simulink library "inp"  (R2021b)
settings: Solver=VariableStepAuto  StartTime=0.0  StopTime=10.0  RelTol=1e-3
undefined symbols (not defined in the file): C_TASK_5MS_S, FALSE, KINP_AcoreReadyToSlp_flg_ovrdflg, KINP_AcoreReadyToSlp_flg_ovrdval, KINP_AllowMovThd_OTA_enum_ovrdflg, KINP_AllowMovThd_OTA_enum_ovrdval, KINP_APSAngleTarget_Deg_ovrdflg, KINP_APSAngleTarget_Deg_ovrdval, KINP_APSDecReq_mps2_ovrdflg, KINP_APSDecReq_mps2_ovrdval, KINP_APSDecReqA_flg_ovrdflg, KINP_APSDecReqA_flg_ovrdval, KINP_APSDFLL_cm_ovrdflg, KINP_APSDFLL_cm_ovrdval, KINP_APSDFLR_cm_ovrdflg, KINP_APSDFLR_cm_ovrdval, KINP_APSDRLL_cm_ovrdflg, KINP_APSDRLL_cm_ovrdval, KINP_APSDRLR_cm_ovrdflg, KINP_APSDRLR_cm_ovrdval, KINP_APSExitCondition_enum_ovrdflg, KINP_APSExitCondition_enum_ovrdval, KINP_APSHWVer_enum_ovrdflg, KINP_APSHWVer_enum_ovrdval, KINP_APSProgressPCT_pct_ovrdflg, KINP_APSProgressPCT_pct_ovrdval, KINP_APSPwrReq_enum_ovrdflg, KINP_APSPwrReq_enum_ovrdval, KINP_APSReq_enum_ovrdflg, KINP_APSReq_enum_ovrdval, KINP_APSRQDisplay_enum_ovrdflg, KINP_APSRQDisplay_enum_ovrdval, KINP_APSRqEPASCtrl_flg_ovrdflg, KINP_APSRqEPASCtrl_flg_ovrdval, KINP_APSShiftPosnReq_enum_ovrdval, KINP_APSShiftPosnReq_enum_ovrflg, KINP_APSSpeedCMD_kph_ovrdval, KINP_APSSpeedCMD_kph_ovrflg, KINP_APSStaSystem_enum_ovrdflg, KINP_APSStaSystem_enum_ovrdval, KINP_APSSWVer_enum_ovrdflg, KINP_APSSWVer_enum_ovrdval, KINP_APSVMCReqA_flg_ovrdval, KINP_APSVMCReqA_flg_ovrflg, KINP_APSVRqEPASCtrl_flg_ovrdflg, KINP_APSVRqEPASCtrl_flg_ovrdval, KINP_AuxBattVolmV_mV_ovrdflg, KINP_AuxBattVolmV_mV_ovrdval, KINP_CAASSta_enum_ovrdflg, KINP_CAASSta_enum_ovrdval, KINP_CAASVMCReqA_flg_ovrdval, KINP_CAASVMCReqA_flg_ovrflg, KINP_CAN1BusOff_flg_ovrdflg, KINP_CAN1BusOff_flg_ovrdval, KINP_CAN2BusOff_flg_ovrdflg, KINP_CAN2BusOff_flg_ovrdval, KINP_CAN3BusOff_flg_ovrdflg, KINP_CAN3BusOff_flg_ovrdval, KINP_CAN4BusOff_flg_ovrdflg, KINP_CAN4BusOff_flg_ovrdval ... (+152)
libraries: FVT_lib x1037, hcu_lib x1
(part 7 of 34)

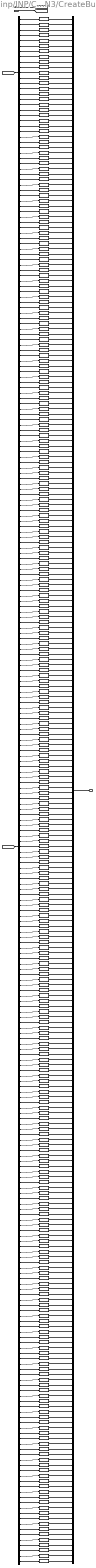
== system inp/INP/CAN3/CreateBus ==
  inp_CanValid_bus : Inport
  inp_Hal_bus : Inport  Port=2
  UnitConverter_{1..23,35,44,63..64,67..75,81..83,87,91..92,102,104..105,107,109,113,115..116,123..125,132..133,135..137,162..164,171..172,174..176,197..201,210..211,213..215,237..238,240..242,251..252,254..256,277..278,283..285,288} (92 alike) : DataTypeConversion  OutDataTypeStr=boolean
  UnitConverter_{26..34,36..43,45..53,58..62,94..97,99..100,110..112,117,126,128..131,139..145,147..148,153..154,161,165,167..170,178..184,186,191..192,202,204,207..209,217..223,225..226,231..232,243,245,248..250,258..266,271..272} (105 alike) : DataTypeConversion  OutDataTypeStr=single
  UnitConverter_{24..25,54..57,65..66,76..80,84..86,88..90,93,98,101,103,106,108,114,118..122,127,134,138,146,149..152,155,158..160,166,173,177,185,187..190,195..196,203,205..206,212,216,224,227..230,233..234,239,244,246..247,253,257,267..270,273..274,279..282,286..287,289..290} (85 alike) : DataTypeConversion  OutDataTypeStr=uint8
  UnitConverter_{156..157,193..194,235..236,275..276} (8 alike) : DataTypeConversion  OutDataTypeStr=uint16
  bus_creator : BusCreator  Inputs=290
  bus_selector : BusSelector  OutputSignals=VINP_CANMsgValidBMS1_flg,VINP_CANMsgValidBMS3_flg,VINP_CANMsgValidBMS4_flg,VINP_CANMsgValidBMS5_flg,VINP_CANMsgValidBMS6_flg,VINP_CANMsgValidBMS8_flg,VINP_CANMsgValidCCU1_flg,VINP_CANMsgValidCCU2_flg,VINP_CANMsgValidEBM1_flg,VINP_CANMsgValidMCUBF1_flg,VINP_CANMsgValidMCUBF2_flg,VINP_CANMsgValidMCUBR1_flg,VINP_CANMsgValidMCUBR2_flg,VINP_CANMsgValidMCUNF1_flg,VINP_CANMsgValidMCUNF2_flg,VINP_CANMsgValidMCUNF3_flg,VINP_CANMsgValidMCUNR1_flg,VINP_CANMsgValidMCUNR2_flg,VINP_CANMsgValidMCUNR3_flg,VINP_CANMsgValidShifter1_flg,VINP_CANMsgValidShifter2_flg
  bus_selector_1 : BusSelector  OutputSignals=VINP_BMS1CSErr_flg,VINP_BMS1RCErr_flg,VINP_BMSChckSum1_enum,VINP_BMSRolCnct1_enum,VINP_HVBPwrAvailChrg_kW,VINP_HVBPwrAvailChrg30_kW,VINP_HVBPwrAvailChrg60_kW,VINP_HVBPwrAvailDchrg_kW,VINP_HVBPwrAvailDchrg30_kW,VINP_HVBPwrAvailDchrg60_kW,VINP_HVBattCurr_A,VINP_HVBattVolt_V,VINP_ACChrgCurrDis_A,VINP_FireDetErr_flg,VINP_HVBChrgPwr_kWh,VINP_HVBChrgPwrTotal_kWh,VINP_HVBDrvPwr_kWh,VINP_HVBDrvPwrTotal_kWh,VINP_HVBFullChrgPwr_kWh,VINP_HVBIsoImpedenceN_Megaohm,VINP_HVBIsoImpedenceP_Megaohm,VINP_HVBSOH_pct,VINP_HVBattErr_flg,VINP_HVBattPackVolt_V,VINP_HVBattSOC_pct,VINP_HVBattSOCDis_pct,VINP_RemainChrgTime_min,VINP_CellTempAvg_C,VINP_HVBCellVoltMax_mV,VINP_HVBCellVoltMin_mV,VINP_HVBMTempMax_C,VINP_HVBMTempMin_C,VINP_MaxCellTempNum_enum,VINP_MaxCellVoltNum_enum,VINP_MinCellTempNum_enum,VINP_MinCellVoltNum_enum,VINP_HVInVolt_V,VINP_LVBattDet12V_V,VINP_OBCACCSLimit_A,VINP_OBCDCCurLm_A,VINP_OBCDCVoltLm_V,VINP_BMS6CSErr_flg,VINP_BMS6RCErr_flg,VINP_BMSChckSum_enum,VINP_BMSRolCnct_enum,VINP_BMSREADY_flg,VINP_BMSWarn1_flg,VINP_BMSWarn2_flg,VINP_BMSWarn3_flg,VINP_BMSWarn4_flg,VINP_BMSWarn5_flg,VINP_BMSWarn6_flg,VINP_BMSWarn7_flg,VINP_BMSWarn8_flg,VINP_ChrgInLockReq_enum,VINP_ChrgPlugSta_enum,VINP_DisChrgPlugErr_enum,VINP_ExtChrgSta_enum,VINP_HVBChrgErr_enum,VINP_HVBContactorSta_flg,VINP_HVBHVILErr_flg,VINP_HVBOvrTempErr_flg,VINP_HVBOvrTempWarn_enum,VINP_HVBPreheatPrecoolSta_enum,VINP_HVBattReady4Pre_enum,VINP_HVILSta_flg,VINP_V2LSta_enum,VINP_MainRlyNegSta_enum,VINP_MainRlyPosSta_enum,VINP_CCU1CSErr_flg,VINP_CCU1RCErr_flg,VINP_CSCCU1_enum,VINP_DCDCAuxCur_A,VINP_DCDCAuxVolt_V,VINP_DCDCHVCur_A,VINP_DCDCInVoltInf_V,VINP_DCDCPreCompleted_enum,VINP_OBCDCCurrInf_A,VINP_OBCDCVoltInf_V,VINP_OBCPreCompleted_enum,VINP_OBCWakeup4Plugin_flg,VINP_RCCCU1_enum,VINP_CCU2CSErr_flg,VINP_CCU2RCErr_flg,VINP_CSCCU2_enum,VINP_DCDCEnaSta_flg,VINP_DCDCFaultSta_enum,VINP_DCDCReady4Pre_flg,VINP_DCDCTemp_C,VINP_OBCACCurrInf_A,VINP_OBCACVoltInf_V,VINP_OBCEnaSta_flg,VINP_OBCFaultSta_enum,VINP_OBCPluginSta_flg,VINP_OBCReady4Pre_flg,VINP_OBCTemp_C,VINP_OBCV2LSta_enum,VINP_OBCACCurLim_enum,VINP_RCCCU2_enum,VINP_EBMErrSta_enum,VINP_EBMRLampSta_enum,VINP_FrActvDmpDisabSta_flg,VINP_FrEDUDrtSta_flg,VINP_FrEDUOpratingSta_flg,VINP_FrEDURealTMTq_Nm,VINP_FrEDURotateDirction_enum,VINP_FrEDUTqReqFbk_Nm,VINP_FrMCUBAT_V,VINP_FrMCUDCBusCurr_A,VINP_FrMCUDCBusVolt_V,VINP_FrMCUDischrgSta_flg,VINP_FrMCUEnaSta_flg,VINP_FrMCUErr_enum,VINP_FrMCUIGNsta_flg,VINP_FrMCUReady_flg,VINP_FrMCUReady4Pre_flg,VINP_FrMCUSysSta_enum,VINP_FrMCUTemp_C,VINP_FrMotorAvailTq_Nm,VINP_FrRegenAvailTq_Nm,VINP_FrTMSpd_rpm,VINP_FrTMTemp_C,VINP_FrTMid_A,VINP_FrTMiq_A,VINP_MCUWarnF_enum,VINP_MCUBFRealPwrKwSta_kW,VINP_FrCoolanttempReq_C,VINP_FrFailcode1_enum,VINP_FrFailcode2_enum,VINP_FrFailcodehistory1_enum,VINP_FrFailcodehistory2_enum,VINP_FrLLCTemp_C,VINP_FrLLCflowReq_Lpmin,VINP_FrMCUTempWarn_enum,VINP_FrMCUHWVer_enum,VINP_FrMCUSWVer_enum,VINP_FrTMTempWarn_enum,VINP_MCUBFLLCTempWarnSta_enum,VINP_MCUWarnR_enum,VINP_MCUBRRealPwrKwSta_kW,VINP_RrActvDmpDisabSta_flg,VINP_RrEDUDrtSta_flg,VINP_RrEDUOpratingSta_flg,VINP_RrEDURealTMTq_Nm,VINP_RrEDURotateDirction_enum,VINP_RrEDUTqReqFbk_Nm,VINP_RrMCUBAT_V,VINP_RrMCUDCBusCurr_A,VINP_RrMCUDCBusVolt_V,VINP_RrMCUDischrgSta_flg,VINP_RrMCUEnaSta_flg,VINP_RrMCUErr_enum,VINP_RrMCUIGNsta_flg,VINP_RrMCUReady_flg,VINP_RrMCUReady4Pre_flg,VINP_RrMCUSysSta_enum,VINP_RrMCUTemp_C,VINP_RrMotorAvailTq_Nm,VINP_RrRegenAvailTq_Nm,VINP_RrTMSpd_rpm,VINP_RrTMTemp_C,VINP_RrTMid_A,VINP_RrTMiq_A,VINP_MCUBRLLCTempWarnSta_enum,VINP_RrCoolanttempReq_cnt,VINP_RrFailcode1_enum,VINP_RrFailcode2_enum,VINP_RrFailcodehistory1_enum,VINP_RrFailcodehistory2_enum,VINP_RrLLCTemp_C,VINP_RrLLCflowReq_Lpmin,VINP_RrMCU3HWVer_enum,VINP_RrMCU3SWVer_enum,VINP_RrMCUTempWarn_enum,VINP_RrTMTempWarn_enum,VINP_MCUNF1CSErr_flg,VINP_MCUNF1RCErr_flg,VINP_FrActvDmpDisabStaNidec_flg,VINP_FrEDUDrtStaNidec_flg,VINP_FrEDUOpratingStaNidec_flg,VINP_FrEDURealTMTqNidec_Nm,VINP_FrEDURotateDirctionNidec_enum,VINP_FrEDUTqReqFbkNidec_Nm,VINP_FrMCU1ChksumNidec_enum,VINP_FrMCU1RolCntNidec_enum,VINP_FrMCUBATNidec_V,VINP_FrMCUDCBusCurrNidec_A,VINP_FrMCUDCBusVoltNidec_V,VINP_FrMCUDischrgStaNidec_flg,VINP_FrMCUEnaStaNidec_flg,VINP_FrMCUErrNidec_enum,VINP_FrMCUIGNstaNidec_flg,VINP_FrMCUReady4PreNidec_flg,VINP_FrMCUReadyNidec_flg,VINP_FrMCUSysStaNidec_enum,VINP_FrMCUTempNidec_C,VINP_FrMotorAvailTqNidec_Nm,VINP_FrRegenAvailTqNidec_Nm,VINP_FrTMSpdNidec_rpm,VINP_FrTMTempNidec_C,VINP_FrTMidNidec_A,VINP_FrTMiqNidec_A,VINP_MCUWarnFNidec_enum,VINP_FrCoolanttempReqNidec_C,VINP_FrEOPSpdSetNidec_rpm,VINP_FrFailcode1Nidec_enum,VINP_FrFailcode2Nidec_enum,VINP_FrFailcodehistory1Nidec_enum,VINP_FrFailcodehistory2Nidec_enum,VINP_FrLLCTempNidec_C,VINP_FrLLCflowReqNidec_Lpmin,VINP_FrMCUTempWarnNidec_enum,VINP_FrTMTempWarnNidec_enum,VINP_FrMCUHWVerNidec_enum,VINP_FrMCUSWVerNidec_enum,VINP_MCUNR1CSErr_flg,VINP_MCUNR1RCErr_flg,VINP_MCUWarnRNidec_enum,VINP_RrActvDmpDisabStaNidec_flg,VINP_RrEDUDrtStaNidec_flg,VINP_RrEDUOpratingStaNidec_flg,VINP_RrEDURealTMTqNidec_Nm,VINP_RrEDURotateDirctionNidec_enum,VINP_RrEDUTqReqFbkNidec_Nm,VINP_RrMCU1ChksumNidec_enum,VINP_RrMCU1RolCntNidec_enum,VINP_RrMCUBATNidec_V,VINP_RrMCUDCBusCurrNidec_A,VINP_RrMCUDCBusVoltNidec_V,VINP_RrMCUDischrgStaNidec_flg,VINP_RrMCUEnaStaNidec_flg,VINP_RrMCUErrNidec_enum,VINP_RrMCUIGNstaNidec_flg,VINP_RrMCUReady4PreNidec_flg,VINP_RrMCUReadyNidec_flg,VINP_RrMCUSysStaNidec_enum,VINP_RrMCUTempNidec_C,VINP_RrMotorAvailTqNidec_Nm,VINP_RrRegenAvailTqNidec_Nm,VINP_RrTMSpdNidec_rpm,VINP_RrTMTempNidec_C,VINP_RrTMidNidec_A,VINP_RrTMiqNidec_A,VINP_RrCoolanttempReqNidec_cnt,VINP_RrEOPSpdSetNidec_rpm,VINP_RrFailcode1Nidec_enum,VINP_RrFailcode2Nidec_enum,VINP_RrFailcodehistory1Nidec_enum,VINP_RrFailcodehistory2Nidec_enum,VINP_RrLLCTempNidec_C,VINP_RrLLCflowReqNidec_Lpmin,VINP_RrMCUTempWarnNidec_enum,VINP_RrTMTempWarnNidec_enum,VINP_RrMCU3HWVerNidec_enum,VINP_RrMCU3SWVerNidec_enum,VINP_Shifter1CSErr_flg,VINP_Shifter1RCErr_flg,VINP_ShifterCRC8_enum,VINP_ShifterFailsta_enum,VINP_ShifterHandleCmd_enum,VINP_ShifterRC_enum,VINP_Shifter2CSErr_flg,VINP_Shifter2RCErr_flg,VINP_CSW2DimSwSta_flg,VINP_CSW2FWasSwSta_enum,VINP_CSW2FWipSwSta_enum,VINP_CSW2PassSWSta_flg,VINP_CSW2RWipWasSwSta_enum,VINP_CSW2TurnSwSta_enum
  BINP_outputs : Outport
  wires:
  inp_CanValid_bus/1 -> [inp_CanValid_bus]
  inp_Hal_bus/1 -> [inp_Hal_bus]
  bus_selector/1 -> UnitConverter_1/1  "<VINP_CANMsgValidBMS1_flg>"
  UnitConverter_1/1 -> bus_creator/1  "VINP_CANMsgValidBMS1_flg"
  bus_selector/2 -> UnitConverter_2/1  "<VINP_CANMsgValidBMS3_flg>"
  UnitConverter_2/1 -> bus_creator/2  "VINP_CANMsgValidBMS3_flg"
  bus_selector/3 -> UnitConverter_3/1  "<VINP_CANMsgValidBMS4_flg>"
  UnitConverter_3/1 -> bus_creator/3  "VINP_CANMsgValidBMS4_flg"
  bus_selector/4 -> UnitConverter_4/1  "<VINP_CANMsgValidBMS5_flg>"
  UnitConverter_4/1 -> bus_creator/4  "VINP_CANMsgValidBMS5_flg"
  bus_selector/5 -> UnitConverter_5/1  "<VINP_CANMsgValidBMS6_flg>"
  UnitConverter_5/1 -> bus_creator/5  "VINP_CANMsgValidBMS6_flg"
  bus_selector/6 -> UnitConverter_6/1  "<VINP_CANMsgValidBMS8_flg>"
  UnitConverter_6/1 -> bus_creator/6  "VINP_CANMsgValidBMS8_flg"
  bus_selector/7 -> UnitConverter_7/1  "<VINP_CANMsgValidCCU1_flg>"
  UnitConverter_7/1 -> bus_creator/7  "VINP_CANMsgValidCCU1_flg"
  bus_selector/8 -> UnitConverter_8/1  "<VINP_CANMsgValidCCU2_flg>"
  UnitConverter_8/1 -> bus_creator/8  "VINP_CANMsgValidCCU2_flg"
  bus_selector/9 -> UnitConverter_9/1  "<VINP_CANMsgValidEBM1_flg>"
  UnitConverter_9/1 -> bus_creator/9  "VINP_CANMsgValidEBM1_flg"
  bus_selector/10 -> UnitConverter_10/1  "<VINP_CANMsgValidMCUBF1_flg>"
  UnitConverter_10/1 -> bus_creator/10  "VINP_CANMsgValidMCUBF1_flg"
  bus_selector/11 -> UnitConverter_11/1  "<VINP_CANMsgValidMCUBF2_flg>"
  UnitConverter_11/1 -> bus_creator/11  "VINP_CANMsgValidMCUBF2_flg"
  bus_selector/12 -> UnitConverter_12/1  "<VINP_CANMsgValidMCUBR1_flg>"
  UnitConverter_12/1 -> bus_creator/12  "VINP_CANMsgValidMCUBR1_flg"
  bus_selector/13 -> UnitConverter_13/1  "<VINP_CANMsgValidMCUBR2_flg>"
  UnitConverter_13/1 -> bus_creator/13  "VINP_CANMsgValidMCUBR2_flg"
  bus_selector/14 -> UnitConverter_14/1  "<VINP_CANMsgValidMCUNF1_flg>"
  UnitConverter_14/1 -> bus_creator/14  "VINP_CANMsgValidMCUNF1_flg"
  bus_selector/15 -> UnitConverter_15/1  "<VINP_CANMsgValidMCUNF2_flg>"
  UnitConverter_15/1 -> bus_creator/15  "VINP_CANMsgValidMCUNF2_flg"
  bus_selector/16 -> UnitConverter_16/1  "<VINP_CANMsgValidMCUNF3_flg>"
  UnitConverter_16/1 -> bus_creator/16  "VINP_CANMsgValidMCUNF3_flg"
  bus_selector/17 -> UnitConverter_17/1  "<VINP_CANMsgValidMCUNR1_flg>"
  UnitConverter_17/1 -> bus_creator/17  "VINP_CANMsgValidMCUNR1_flg"
  bus_selector/18 -> UnitConverter_18/1  "<VINP_CANMsgValidMCUNR2_flg>"
  UnitConverter_18/1 -> bus_creator/18  "VINP_CANMsgValidMCUNR2_flg"
  bus_selector/19 -> UnitConverter_19/1  "<VINP_CANMsgValidMCUNR3_flg>"
  UnitConverter_19/1 -> bus_creator/19  "VINP_CANMsgValidMCUNR3_flg"
  bus_selector/20 -> UnitConverter_20/1  "<VINP_CANMsgValidShifter1_flg>"
  UnitConverter_20/1 -> bus_creator/20  "VINP_CANMsgValidShifter1_flg"
  bus_selector/21 -> UnitConverter_21/1  "<VINP_CANMsgValidShifter2_flg>"
  UnitConverter_21/1 -> bus_creator/21  "VINP_CANMsgValidShifter2_flg"
  bus_selector_1/1 -> UnitConverter_22/1  "<VINP_BMS1CSErr_flg>"
  UnitConverter_22/1 -> bus_creator/22  "VINP_BMS1CSErr_flg"
  bus_selector_1/2 -> UnitConverter_23/1  "<VINP_BMS1RCErr_flg>"
  UnitConverter_23/1 -> bus_creator/23  "VINP_BMS1RCErr_flg"
  bus_selector_1/3 -> UnitConverter_24/1  "<VINP_BMSChckSum1_enum>"
  UnitConverter_24/1 -> bus_creator/24  "VINP_BMSChckSum1_enum"
  bus_selector_1/4 -> UnitConverter_25/1  "<VINP_BMSRolCnct1_enum>"
  UnitConverter_25/1 -> bus_creator/25  "VINP_BMSRolCnct1_enum"
  bus_selector_1/5 -> UnitConverter_26/1  "<VINP_HVBPwrAvailChrg_kW>"
  UnitConverter_26/1 -> bus_creator/26  "VINP_HVBPwrAvailChrg_kW"
  bus_selector_1/6 -> UnitConverter_27/1  "<VINP_HVBPwrAvailChrg30_kW>"
  UnitConverter_27/1 -> bus_creator/27  "VINP_HVBPwrAvailChrg30_kW"
  bus_selector_1/7 -> UnitConverter_28/1  "<VINP_HVBPwrAvailChrg60_kW>"
  UnitConverter_28/1 -> bus_creator/28  "VINP_HVBPwrAvailChrg60_kW"
  bus_selector_1/8 -> UnitConverter_29/1  "<VINP_HVBPwrAvailDchrg_kW>"
  UnitConverter_29/1 -> bus_creator/29  "VINP_HVBPwrAvailDchrg_kW"
  bus_selector_1/9 -> UnitConverter_30/1  "<VINP_HVBPwrAvailDchrg30_kW>"
  UnitConverter_30/1 -> bus_creator/30  "VINP_HVBPwrAvailDchrg30_kW"
  bus_selector_1/10 -> UnitConverter_31/1  "<VINP_HVBPwrAvailDchrg60_kW>"
  UnitConverter_31/1 -> bus_creator/31  "VINP_HVBPwrAvailDchrg60_kW"
  bus_selector_1/11 -> UnitConverter_32/1  "<VINP_HVBattCurr_A>"
  UnitConverter_32/1 -> bus_creator/32  "VINP_HVBattCurr_A"
  bus_selector_1/12 -> UnitConverter_33/1  "<VINP_HVBattVolt_V>"
  UnitConverter_33/1 -> bus_creator/33  "VINP_HVBattVolt_V"
  bus_selector_1/13 -> UnitConverter_34/1  "<VINP_ACChrgCurrDis_A>"
  UnitConverter_34/1 -> bus_creator/34  "VINP_ACChrgCurrDis_A"
  bus_selector_1/14 -> UnitConverter_35/1  "<VINP_FireDetErr_flg>"
  UnitConverter_35/1 -> bus_creator/35  "VINP_FireDetErr_flg"
  bus_selector_1/15 -> UnitConverter_36/1  "<VINP_HVBChrgPwr_kWh>"
  UnitConverter_36/1 -> bus_creator/36  "VINP_HVBChrgPwr_kWh"
  bus_selector_1/16 -> UnitConverter_37/1  "<VINP_HVBChrgPwrTotal_kWh>"
  UnitConverter_37/1 -> bus_creator/37  "VINP_HVBChrgPwrTotal_kWh"
  bus_selector_1/17 -> UnitConverter_38/1  "<VINP_HVBDrvPwr_kWh>"
  UnitConverter_38/1 -> bus_creator/38  "VINP_HVBDrvPwr_kWh"
  bus_selector_1/18 -> UnitConverter_39/1  "<VINP_HVBDrvPwrTotal_kWh>"
  UnitConverter_39/1 -> bus_creator/39  "VINP_HVBDrvPwrTotal_kWh"
  bus_selector_1/19 -> UnitConverter_40/1  "<VINP_HVBFullChrgPwr_kWh>"
  UnitConverter_40/1 -> bus_creator/40  "VINP_HVBFullChrgPwr_kWh"
  bus_selector_1/20 -> UnitConverter_41/1  "<VINP_HVBIsoImpedenceN_Megaohm>"
  UnitConverter_41/1 -> bus_creator/41  "VINP_HVBIsoImpedenceN_Megaohm"
  bus_selector_1/21 -> UnitConverter_42/1  "<VINP_HVBIsoImpedenceP_Megaohm>"
  UnitConverter_42/1 -> bus_creator/42  "VINP_HVBIsoImpedenceP_Megaohm"
  bus_selector_1/22 -> UnitConverter_43/1  "<VINP_HVBSOH_pct>"
  UnitConverter_43/1 -> bus_creator/43  "VINP_HVBSOH_pct"
  bus_selector_1/23 -> UnitConverter_44/1  "<VINP_HVBattErr_flg>"
  UnitConverter_44/1 -> bus_creator/44  "VINP_HVBattErr_flg"
  bus_selector_1/24 -> UnitConverter_45/1  "<VINP_HVBattPackVolt_V>"
  UnitConverter_45/1 -> bus_creator/45  "VINP_HVBattPackVolt_V"
  bus_selector_1/25 -> UnitConverter_46/1  "<VINP_HVBattSOC_pct>"
  UnitConverter_46/1 -> bus_creator/46  "VINP_HVBattSOC_pct"
  bus_selector_1/26 -> UnitConverter_47/1  "<VINP_HVBattSOCDis_pct>"
  UnitConverter_47/1 -> bus_creator/47  "VINP_HVBattSOCDis_pct"
  bus_selector_1/27 -> UnitConverter_48/1  "<VINP_RemainChrgTime_min>"
  UnitConverter_48/1 -> bus_creator/48  "VINP_RemainChrgTime_min"
  bus_selector_1/28 -> UnitConverter_49/1  "<VINP_CellTempAvg_C>"
  UnitConverter_49/1 -> bus_creator/49  "VINP_CellTempAvg_C"
  bus_selector_1/29 -> UnitConverter_50/1  "<VINP_HVBCellVoltMax_mV>"
  UnitConverter_50/1 -> bus_creator/50  "VINP_HVBCellVoltMax_mV"
  bus_selector_1/30 -> UnitConverter_51/1  "<VINP_HVBCellVoltMin_mV>"
  UnitConverter_51/1 -> bus_creator/51  "VINP_HVBCellVoltMin_mV"
  bus_selector_1/31 -> UnitConverter_52/1  "<VINP_HVBMTempMax_C>"
  UnitConverter_52/1 -> bus_creator/52  "VINP_HVBMTempMax_C"
  bus_selector_1/32 -> UnitConverter_53/1  "<VINP_HVBMTempMin_C>"
  UnitConverter_53/1 -> bus_creator/53  "VINP_HVBMTempMin_C"
  bus_selector_1/33 -> UnitConverter_54/1  "<VINP_MaxCellTempNum_enum>"
  UnitConverter_54/1 -> bus_creator/54  "VINP_MaxCellTempNum_enum"
  bus_selector_1/34 -> UnitConverter_55/1  "<VINP_MaxCellVoltNum_enum>"
  UnitConverter_55/1 -> bus_creator/55  "VINP_MaxCellVoltNum_enum"
  bus_selector_1/35 -> UnitConverter_56/1  "<VINP_MinCellTempNum_enum>"
  UnitConverter_56/1 -> bus_creator/56  "VINP_MinCellTempNum_enum"
  bus_selector_1/36 -> UnitConverter_57/1  "<VINP_MinCellVoltNum_enum>"
  UnitConverter_57/1 -> bus_creator/57  "VINP_MinCellVoltNum_enum"
  bus_selector_1/37 -> UnitConverter_58/1  "<VINP_HVInVolt_V>"
  UnitConverter_58/1 -> bus_creator/58  "VINP_HVInVolt_V"
  bus_selector_1/38 -> UnitConverter_59/1  "<VINP_LVBattDet12V_V>"
  UnitConverter_59/1 -> bus_creator/59  "VINP_LVBattDet12V_V"
  bus_selector_1/39 -> UnitConverter_60/1  "<VINP_OBCACCSLimit_A>"
  UnitConverter_60/1 -> bus_creator/60  "VINP_OBCACCSLimit_A"
  bus_selector_1/40 -> UnitConverter_61/1  "<VINP_OBCDCCurLm_A>"
  UnitConverter_61/1 -> bus_creator/61  "VINP_OBCDCCurLm_A"
  bus_selector_1/41 -> UnitConverter_62/1  "<VINP_OBCDCVoltLm_V>"
  UnitConverter_62/1 -> bus_creator/62  "VINP_OBCDCVoltLm_V"
  bus_selector_1/42 -> UnitConverter_63/1  "<VINP_BMS6CSErr_flg>"
  UnitConverter_63/1 -> bus_creator/63  "VINP_BMS6CSErr_flg"
  bus_selector_1/43 -> UnitConverter_64/1  "<VINP_BMS6RCErr_flg>"
  UnitConverter_64/1 -> bus_creator/64  "VINP_BMS6RCErr_flg"
  bus_selector_1/44 -> UnitConverter_65/1  "<VINP_BMSChckSum_enum>"
  UnitConverter_65/1 -> bus_creator/65  "VINP_BMSChckSum_enum"
  bus_selector_1/45 -> UnitConverter_66/1  "<VINP_BMSRolCnct_enum>"
  UnitConverter_66/1 -> bus_creator/66  "VINP_BMSRolCnct_enum"
  bus_selector_1/46 -> UnitConverter_67/1  "<VINP_BMSREADY_flg>"
  UnitConverter_67/1 -> bus_creator/67  "VINP_BMSREADY_flg"
  bus_selector_1/47 -> UnitConverter_68/1  "<VINP_BMSWarn1_flg>"
  UnitConverter_68/1 -> bus_creator/68  "VINP_BMSWarn1_flg"
  bus_selector_1/48 -> UnitConverter_69/1  "<VINP_BMSWarn2_flg>"
  UnitConverter_69/1 -> bus_creator/69  "VINP_BMSWarn2_flg"
  bus_selector_1/49 -> UnitConverter_70/1  "<VINP_BMSWarn3_flg>"
  UnitConverter_70/1 -> bus_creator/70  "VINP_BMSWarn3_flg"
  bus_selector_1/50 -> UnitConverter_71/1  "<VINP_BMSWarn4_flg>"
  UnitConverter_71/1 -> bus_creator/71  "VINP_BMSWarn4_flg"
  bus_selector_1/51 -> UnitConverter_72/1  "<VINP_BMSWarn5_flg>"
  UnitConverter_72/1 -> bus_creator/72  "VINP_BMSWarn5_flg"
  bus_selector_1/52 -> UnitConverter_73/1  "<VINP_BMSWarn6_flg>"
  UnitConverter_73/1 -> bus_creator/73  "VINP_BMSWarn6_flg"
  bus_selector_1/53 -> UnitConverter_74/1  "<VINP_BMSWarn7_flg>"
  UnitConverter_74/1 -> bus_creator/74  "VINP_BMSWarn7_flg"
  bus_selector_1/54 -> UnitConverter_75/1  "<VINP_BMSWarn8_flg>"
  UnitConverter_75/1 -> bus_creator/75  "VINP_BMSWarn8_flg"
  bus_selector_1/55 -> UnitConverter_76/1  "<VINP_ChrgInLockReq_enum>"
  UnitConverter_76/1 -> bus_creator/76  "VINP_ChrgInLockReq_enum"
  bus_selector_1/56 -> UnitConverter_77/1  "<VINP_ChrgPlugSta_enum>"
  UnitConverter_77/1 -> bus_creator/77  "VINP_ChrgPlugSta_enum"
  bus_selector_1/57 -> UnitConverter_78/1  "<VINP_DisChrgPlugErr_enum>"
  UnitConverter_78/1 -> bus_creator/78  "VINP_DisChrgPlugErr_enum"
  bus_selector_1/58 -> UnitConverter_79/1  "<VINP_ExtChrgSta_enum>"
  UnitConverter_79/1 -> bus_creator/79  "VINP_ExtChrgSta_enum"
  bus_selector_1/59 -> UnitConverter_80/1  "<VINP_HVBChrgErr_enum>"
  UnitConverter_80/1 -> bus_creator/80  "VINP_HVBChrgErr_enum"
  bus_selector_1/60 -> UnitConverter_81/1  "<VINP_HVBContactorSta_flg>"
  UnitConverter_81/1 -> bus_creator/81  "VINP_HVBContactorSta_flg"
  bus_selector_1/61 -> UnitConverter_82/1  "<VINP_HVBHVILErr_flg>"
  UnitConverter_82/1 -> bus_creator/82  "VINP_HVBHVILErr_flg"
  bus_selector_1/62 -> UnitConverter_83/1  "<VINP_HVBOvrTempErr_flg>"
  UnitConverter_83/1 -> bus_creator/83  "VINP_HVBOvrTempErr_flg"
  bus_selector_1/63 -> UnitConverter_84/1  "<VINP_HVBOvrTempWarn_enum>"
  UnitConverter_84/1 -> bus_creator/84  "VINP_HVBOvrTempWarn_enum"
  bus_selector_1/64 -> UnitConverter_85/1  "<VINP_HVBPreheatPrecoolSta_enum>"
  UnitConverter_85/1 -> bus_creator/85  "VINP_HVBPreheatPrecoolSta_enum"
  bus_selector_1/65 -> UnitConverter_86/1  "<VINP_HVBattReady4Pre_enum>"
  UnitConverter_86/1 -> bus_creator/86  "VINP_HVBattReady4Pre_enum"
  bus_selector_1/66 -> UnitConverter_87/1  "<VINP_HVILSta_flg>"
  UnitConverter_87/1 -> bus_creator/87  "VINP_HVILSta_flg"
  bus_selector_1/67 -> UnitConverter_88/1  "<VINP_V2LSta_enum>"
  UnitConverter_88/1 -> bus_creator/88  "VINP_V2LSta_enum"
  bus_selector_1/68 -> UnitConverter_89/1  "<VINP_MainRlyNegSta_enum>"
  UnitConverter_89/1 -> bus_creator/89  "VINP_MainRlyNegSta_enum"
  bus_selector_1/69 -> UnitConverter_90/1  "<VINP_MainRlyPosSta_enum>"
  UnitConverter_90/1 -> bus_creator/90  "VINP_MainRlyPosSta_enum"
  bus_selector_1/70 -> UnitConverter_91/1  "<VINP_CCU1CSErr_flg>"
  UnitConverter_91/1 -> bus_creator/91  "VINP_CCU1CSErr_flg"
  bus_selector_1/71 -> UnitConverter_92/1  "<VINP_CCU1RCErr_flg>"
  UnitConverter_92/1 -> bus_creator/92  "VINP_CCU1RCErr_flg"
  bus_selector_1/72 -> UnitConverter_93/1  "<VINP_CSCCU1_enum>"
  UnitConverter_93/1 -> bus_creator/93  "VINP_CSCCU1_enum"
  bus_selector_1/73 -> UnitConverter_94/1  "<VINP_DCDCAuxCur_A>"
  UnitConverter_94/1 -> bus_creator/94  "VINP_DCDCAuxCur_A"
  bus_selector_1/74 -> UnitConverter_95/1  "<VINP_DCDCAuxVolt_V>"
  UnitConverter_95/1 -> bus_creator/95  "VINP_DCDCAuxVolt_V"
  bus_selector_1/75 -> UnitConverter_96/1  "<VINP_DCDCHVCur_A>"
  UnitConverter_96/1 -> bus_creator/96  "VINP_DCDCHVCur_A"
  bus_selector_1/76 -> UnitConverter_97/1  "<VINP_DCDCInVoltInf_V>"
  UnitConverter_97/1 -> bus_creator/97  "VINP_DCDCInVoltInf_V"
  bus_selector_1/77 -> UnitConverter_98/1  "<VINP_DCDCPreCompleted_enum>"
  UnitConverter_98/1 -> bus_creator/98  "VINP_DCDCPreCompleted_enum"
  bus_selector_1/78 -> UnitConverter_99/1  "<VINP_OBCDCCurrInf_A>"
  UnitConverter_99/1 -> bus_creator/99  "VINP_OBCDCCurrInf_A"
  bus_selector_1/79 -> UnitConverter_100/1  "<VINP_OBCDCVoltInf_V>"
  UnitConverter_100/1 -> bus_creator/100  "VINP_OBCDCVoltInf_V"
  bus_selector_1/80 -> UnitConverter_101/1  "<VINP_OBCPreCompleted_enum>"
  UnitConverter_101/1 -> bus_creator/101  "VINP_OBCPreCompleted_enum"
  bus_selector_1/81 -> UnitConverter_102/1  "<VINP_OBCWakeup4Plugin_flg>"
  UnitConverter_102/1 -> bus_creator/102  "VINP_OBCWakeup4Plugin_flg"
  bus_selector_1/82 -> UnitConverter_103/1  "<VINP_RCCCU1_enum>"
  UnitConverter_103/1 -> bus_creator/103  "VINP_RCCCU1_enum"
  bus_selector_1/83 -> UnitConverter_104/1  "<VINP_CCU2CSErr_flg>"
  UnitConverter_104/1 -> bus_creator/104  "VINP_CCU2CSErr_flg"
  bus_selector_1/84 -> UnitConverter_105/1  "<VINP_CCU2RCErr_flg>"
  UnitConverter_105/1 -> bus_creator/105  "VINP_CCU2RCErr_flg"
  bus_selector_1/85 -> UnitConverter_106/1  "<VINP_CSCCU2_enum>"
  UnitConverter_106/1 -> bus_creator/106  "VINP_CSCCU2_enum"
  bus_selector_1/86 -> UnitConverter_107/1  "<VINP_DCDCEnaSta_flg>"
  UnitConverter_107/1 -> bus_creator/107  "VINP_DCDCEnaSta_flg"
  bus_selector_1/87 -> UnitConverter_108/1  "<VINP_DCDCFaultSta_enum>"
  UnitConverter_108/1 -> bus_creator/108  "VINP_DCDCFaultSta_enum"
  bus_selector_1/88 -> UnitConverter_109/1  "<VINP_DCDCReady4Pre_flg>"
  UnitConverter_109/1 -> bus_creator/109  "VINP_DCDCReady4Pre_flg"
  bus_selector_1/89 -> UnitConverter_110/1  "<VINP_DCDCTemp_C>"
  UnitConverter_110/1 -> bus_creator/110  "VINP_DCDCTemp_C"
  bus_selector_1/90 -> UnitConverter_111/1  "<VINP_OBCACCurrInf_A>"
  UnitConverter_111/1 -> bus_creator/111  "VINP_OBCACCurrInf_A"
  bus_selector_1/91 -> UnitConverter_112/1  "<VINP_OBCACVoltInf_V>"
  UnitConverter_112/1 -> bus_creator/112  "VINP_OBCACVoltInf_V"
  bus_selector_1/92 -> UnitConverter_113/1  "<VINP_OBCEnaSta_flg>"
  UnitConverter_113/1 -> bus_creator/113  "VINP_OBCEnaSta_flg"
  bus_selector_1/93 -> UnitConverter_114/1  "<VINP_OBCFaultSta_enum>"
  UnitConverter_114/1 -> bus_creator/114  "VINP_OBCFaultSta_enum"
  bus_selector_1/94 -> UnitConverter_115/1  "<VINP_OBCPluginSta_flg>"
  UnitConverter_115/1 -> bus_creator/115  "VINP_OBCPluginSta_flg"
  bus_selector_1/95 -> UnitConverter_116/1  "<VINP_OBCReady4Pre_flg>"
  UnitConverter_116/1 -> bus_creator/116  "VINP_OBCReady4Pre_flg"
  bus_selector_1/96 -> UnitConverter_117/1  "<VINP_OBCTemp_C>"
  UnitConverter_117/1 -> bus_creator/117  "VINP_OBCTemp_C"
  bus_selector_1/97 -> UnitConverter_118/1  "<VINP_OBCV2LSta_enum>"
  UnitConverter_118/1 -> bus_creator/118  "VINP_OBCV2LSta_enum"
  bus_selector_1/98 -> UnitConverter_119/1  "<VINP_OBCACCurLim_enum>"
  UnitConverter_119/1 -> bus_creator/119  "VINP_OBCACCurLim_enum"
  bus_selector_1/99 -> UnitConverter_120/1  "<VINP_RCCCU2_enum>"
  UnitConverter_120/1 -> bus_creator/120  "VINP_RCCCU2_enum"
  bus_selector_1/100 -> UnitConverter_121/1  "<VINP_EBMErrSta_enum>"
  UnitConverter_121/1 -> bus_creator/121  "VINP_EBMErrSta_enum"
  bus_selector_1/101 -> UnitConverter_122/1  "<VINP_EBMRLampSta_enum>"
  UnitConverter_122/1 -> bus_creator/122  "VINP_EBMRLampSta_enum"
  bus_selector_1/102 -> UnitConverter_123/1  "<VINP_FrActvDmpDisabSta_flg>"
  UnitConverter_123/1 -> bus_creator/123  "VINP_FrActvDmpDisabSta_flg"
  bus_selector_1/103 -> UnitConverter_124/1  "<VINP_FrEDUDrtSta_flg>"
  UnitConverter_124/1 -> bus_creator/124  "VINP_FrEDUDrtSta_flg"
  bus_selector_1/104 -> UnitConverter_125/1  "<VINP_FrEDUOpratingSta_flg>"
  UnitConverter_125/1 -> bus_creator/125  "VINP_FrEDUOpratingSta_flg"
  bus_selector_1/105 -> UnitConverter_126/1  "<VINP_FrEDURealTMTq_Nm>"
  UnitConverter_126/1 -> bus_creator/126  "VINP_FrEDURealTMTq_Nm"
  bus_selector_1/106 -> UnitConverter_127/1  "<VINP_FrEDURotateDirction_enum>"
  UnitConverter_127/1 -> bus_creator/127  "VINP_FrEDURotateDirction_enum"
  bus_selector_1/107 -> UnitConverter_128/1  "<VINP_FrEDUTqReqFbk_Nm>"
  UnitConverter_128/1 -> bus_creator/128  "VINP_FrEDUTqReqFbk_Nm"
  bus_selector_1/108 -> UnitConverter_129/1  "<VINP_FrMCUBAT_V>"
  UnitConverter_129/1 -> bus_creator/129  "VINP_FrMCUBAT_V"
  bus_selector_1/109 -> UnitConverter_130/1  "<VINP_FrMCUDCBusCurr_A>"
  UnitConverter_130/1 -> bus_creator/130  "VINP_FrMCUDCBusCurr_A"
  bus_selector_1/110 -> UnitConverter_131/1  "<VINP_FrMCUDCBusVolt_V>"
  UnitConverter_131/1 -> bus_creator/131  "VINP_FrMCUDCBusVolt_V"
  bus_selector_1/111 -> UnitConverter_132/1  "<VINP_FrMCUDischrgSta_flg>"
  UnitConverter_132/1 -> bus_creator/132  "VINP_FrMCUDischrgSta_flg"
  bus_selector_1/112 -> UnitConverter_133/1  "<VINP_FrMCUEnaSta_flg>"
  UnitConverter_133/1 -> bus_creator/133  "VINP_FrMCUEnaSta_flg"
  bus_selector_1/113 -> UnitConverter_134/1  "<VINP_FrMCUErr_enum>"
  UnitConverter_134/1 -> bus_creator/134  "VINP_FrMCUErr_enum"
  bus_selector_1/114 -> UnitConverter_135/1  "<VINP_FrMCUIGNsta_flg>"
  UnitConverter_135/1 -> bus_creator/135  "VINP_FrMCUIGNsta_flg"
  bus_selector_1/115 -> UnitConverter_136/1  "<VINP_FrMCUReady_flg>"
  UnitConverter_136/1 -> bus_creator/136  "VINP_FrMCUReady_flg"
  bus_selector_1/116 -> UnitConverter_137/1  "<VINP_FrMCUReady4Pre_flg>"
  UnitConverter_137/1 -> bus_creator/137  "VINP_FrMCUReady4Pre_flg"
  bus_selector_1/117 -> UnitConverter_138/1  "<VINP_FrMCUSysSta_enum>"
  UnitConverter_138/1 -> bus_creator/138  "VINP_FrMCUSysSta_enum"
  bus_selector_1/118 -> UnitConverter_139/1  "<VINP_FrMCUTemp_C>"
  UnitConverter_139/1 -> bus_creator/139  "VINP_FrMCUTemp_C"
  bus_selector_1/119 -> UnitConverter_140/1  "<VINP_FrMotorAvailTq_Nm>"
  UnitConverter_140/1 -> bus_creator/140  "VINP_FrMotorAvailTq_Nm"
  bus_selector_1/120 -> UnitConverter_141/1  "<VINP_FrRegenAvailTq_Nm>"
  UnitConverter_141/1 -> bus_creator/141  "VINP_FrRegenAvailTq_Nm"
  bus_selector_1/121 -> UnitConverter_142/1  "<VINP_FrTMSpd_rpm>"
  UnitConverter_142/1 -> bus_creator/142  "VINP_FrTMSpd_rpm"
  bus_selector_1/122 -> UnitConverter_143/1  "<VINP_FrTMTemp_C>"
  UnitConverter_143/1 -> bus_creator/143  "VINP_FrTMTemp_C"
  bus_selector_1/123 -> UnitConverter_144/1  "<VINP_FrTMid_A>"
  UnitConverter_144/1 -> bus_creator/144  "VINP_FrTMid_A"
  bus_selector_1/124 -> UnitConverter_145/1  "<VINP_FrTMiq_A>"
  UnitConverter_145/1 -> bus_creator/145  "VINP_FrTMiq_A"
  bus_selector_1/125 -> UnitConverter_146/1  "<VINP_MCUWarnF_enum>"
  UnitConverter_146/1 -> bus_creator/146  "VINP_MCUWarnF_enum"
  bus_selector_1/126 -> UnitConverter_147/1  "<VINP_MCUBFRealPwrKwSta_kW>"
  UnitConverter_147/1 -> bus_creator/147  "VINP_MCUBFRealPwrKwSta_kW"
  bus_selector_1/127 -> UnitConverter_148/1  "<VINP_FrCoolanttempReq_C>"
  UnitConverter_148/1 -> bus_creator/148  "VINP_FrCoolanttempReq_C"
  bus_selector_1/128 -> UnitConverter_149/1  "<VINP_FrFailcode1_enum>"
  UnitConverter_149/1 -> bus_creator/149  "VINP_FrFailcode1_enum"
  bus_selector_1/129 -> UnitConverter_150/1  "<VINP_FrFailcode2_enum>"
  UnitConverter_150/1 -> bus_creator/150  "VINP_FrFailcode2_enum"
  bus_selector_1/130 -> UnitConverter_151/1  "<VINP_FrFailcodehistory1_enum>"
  UnitConverter_151/1 -> bus_creator/151  "VINP_FrFailcodehistory1_enum"
  bus_selector_1/131 -> UnitConverter_152/1  "<VINP_FrFailcodehistory2_enum>"
  UnitConverter_152/1 -> bus_creator/152  "VINP_FrFailcodehistory2_enum"
  bus_selector_1/132 -> UnitConverter_153/1  "<VINP_FrLLCTemp_C>"
  UnitConverter_153/1 -> bus_creator/153  "VINP_FrLLCTemp_C"
  bus_selector_1/133 -> UnitConverter_154/1  "<VINP_FrLLCflowReq_Lpmin>"
  UnitConverter_154/1 -> bus_creator/154  "VINP_FrLLCflowReq_Lpmin"
  bus_selector_1/134 -> UnitConverter_155/1  "<VINP_FrMCUTempWarn_enum>"
  UnitConverter_155/1 -> bus_creator/155  "VINP_FrMCUTempWarn_enum"
  bus_selector_1/135 -> UnitConverter_156/1  "<VINP_FrMCUHWVer_enum>"
  UnitConverter_156/1 -> bus_creator/156  "VINP_FrMCUHWVer_enum"
  bus_selector_1/136 -> UnitConverter_157/1  "<VINP_FrMCUSWVer_enum>"
  UnitConverter_157/1 -> bus_creator/157  "VINP_FrMCUSWVer_enum"
  bus_selector_1/137 -> UnitConverter_158/1  "<VINP_FrTMTempWarn_enum>"
  UnitConverter_158/1 -> bus_creator/158  "VINP_FrTMTempWarn_enum"
  bus_selector_1/138 -> UnitConverter_159/1  "<VINP_MCUBFLLCTempWarnSta_enum>"
  UnitConverter_159/1 -> bus_creator/159  "VINP_MCUBFLLCTempWarnSta_enum"
  bus_selector_1/139 -> UnitConverter_160/1  "<VINP_MCUWarnR_enum>"
  UnitConverter_160/1 -> bus_creator/160  "VINP_MCUWarnR_enum"
  bus_selector_1/140 -> UnitConverter_161/1  "<VINP_MCUBRRealPwrKwSta_kW>"
  UnitConverter_161/1 -> bus_creator/161  "VINP_MCUBRRealPwrKwSta_kW"
  bus_selector_1/141 -> UnitConverter_162/1  "<VINP_RrActvDmpDisabSta_flg>"
  UnitConverter_162/1 -> bus_creator/162  "VINP_RrActvDmpDisabSta_flg"
  bus_selector_1/142 -> UnitConverter_163/1  "<VINP_RrEDUDrtSta_flg>"
  UnitConverter_163/1 -> bus_creator/163  "VINP_RrEDUDrtSta_flg"
  bus_selector_1/143 -> UnitConverter_164/1  "<VINP_RrEDUOpratingSta_flg>"
  UnitConverter_164/1 -> bus_creator/164  "VINP_RrEDUOpratingSta_flg"
  bus_selector_1/144 -> UnitConverter_165/1  "<VINP_RrEDURealTMTq_Nm>"
  UnitConverter_165/1 -> bus_creator/165  "VINP_RrEDURealTMTq_Nm"
  bus_selector_1/145 -> UnitConverter_166/1  "<VINP_RrEDURotateDirction_enum>"
  UnitConverter_166/1 -> bus_creator/166  "VINP_RrEDURotateDirction_enum"
  bus_selector_1/146 -> UnitConverter_167/1  "<VINP_RrEDUTqReqFbk_Nm>"
  UnitConverter_167/1 -> bus_creator/167  "VINP_RrEDUTqReqFbk_Nm"
  bus_selector_1/147 -> UnitConverter_168/1  "<VINP_RrMCUBAT_V>"
  UnitConverter_168/1 -> bus_creator/168  "VINP_RrMCUBAT_V"
  bus_selector_1/148 -> UnitConverter_169/1  "<VINP_RrMCUDCBusCurr_A>"
  UnitConverter_169/1 -> bus_creator/169  "VINP_RrMCUDCBusCurr_A"
  bus_selector_1/149 -> UnitConverter_170/1  "<VINP_RrMCUDCBusVolt_V>"
  UnitConverter_170/1 -> bus_creator/170  "VINP_RrMCUDCBusVolt_V"
  bus_selector_1/150 -> UnitConverter_171/1  "<VINP_RrMCUDischrgSta_flg>"
  UnitConverter_171/1 -> bus_creator/171  "VINP_RrMCUDischrgSta_flg"
  bus_selector_1/151 -> UnitConverter_172/1  "<VINP_RrMCUEnaSta_flg>"
  UnitConverter_172/1 -> bus_creator/172  "VINP_RrMCUEnaSta_flg"
  bus_selector_1/152 -> UnitConverter_173/1  "<VINP_RrMCUErr_enum>"
  UnitConverter_173/1 -> bus_creator/173  "VINP_RrMCUErr_enum"
  bus_selector_1/153 -> UnitConverter_174/1  "<VINP_RrMCUIGNsta_flg>"
  UnitConverter_174/1 -> bus_creator/174  "VINP_RrMCUIGNsta_flg"
  bus_selector_1/154 -> UnitConverter_175/1  "<VINP_RrMCUReady_flg>"
  UnitConverter_175/1 -> bus_creator/175  "VINP_RrMCUReady_flg"
  bus_selector_1/155 -> UnitConverter_176/1  "<VINP_RrMCUReady4Pre_flg>"
  UnitConverter_176/1 -> bus_creator/176  "VINP_RrMCUReady4Pre_flg"
  bus_selector_1/156 -> UnitConverter_177/1  "<VINP_RrMCUSysSta_enum>"
  UnitConverter_177/1 -> bus_creator/177  "VINP_RrMCUSysSta_enum"
  bus_selector_1/157 -> UnitConverter_178/1  "<VINP_RrMCUTemp_C>"
  UnitConverter_178/1 -> bus_creator/178  "VINP_RrMCUTemp_C"
  bus_selector_1/158 -> UnitConverter_179/1  "<VINP_RrMotorAvailTq_Nm>"
  UnitConverter_179/1 -> bus_creator/179  "VINP_RrMotorAvailTq_Nm"
  bus_selector_1/159 -> UnitConverter_180/1  "<VINP_RrRegenAvailTq_Nm>"
  UnitConverter_180/1 -> bus_creator/180  "VINP_RrRegenAvailTq_Nm"
  bus_selector_1/160 -> UnitConverter_181/1  "<VINP_RrTMSpd_rpm>"
  UnitConverter_181/1 -> bus_creator/181  "VINP_RrTMSpd_rpm"
  bus_selector_1/161 -> UnitConverter_182/1  "<VINP_RrTMTemp_C>"
  UnitConverter_182/1 -> bus_creator/182  "VINP_RrTMTemp_C"
  bus_selector_1/162 -> UnitConverter_183/1  "<VINP_RrTMid_A>"
  UnitConverter_183/1 -> bus_creator/183  "VINP_RrTMid_A"
  bus_selector_1/163 -> UnitConverter_184/1  "<VINP_RrTMiq_A>"
  UnitConverter_184/1 -> bus_creator/184  "VINP_RrTMiq_A"
  bus_selector_1/164 -> UnitConverter_185/1  "<VINP_MCUBRLLCTempWarnSta_enum>"
  UnitConverter_185/1 -> bus_creator/185  "VINP_MCUBRLLCTempWarnSta_enum"
  bus_selector_1/165 -> UnitConverter_186/1  "<VINP_RrCoolanttempReq_cnt>"
  UnitConverter_186/1 -> bus_creator/186  "VINP_RrCoolanttempReq_cnt"
  bus_selector_1/166 -> UnitConverter_187/1  "<VINP_RrFailcode1_enum>"
  UnitConverter_187/1 -> bus_creator/187  "VINP_RrFailcode1_enum"
  bus_selector_1/167 -> UnitConverter_188/1  "<VINP_RrFailcode2_enum>"
  UnitConverter_188/1 -> bus_creator/188  "VINP_RrFailcode2_enum"
  bus_selector_1/168 -> UnitConverter_189/1  "<VINP_RrFailcodehistory1_enum>"
  UnitConverter_189/1 -> bus_creator/189  "VINP_RrFailcodehistory1_enum"
  bus_selector_1/169 -> UnitConverter_190/1  "<VINP_RrFailcodehistory2_enum>"
  UnitConverter_190/1 -> bus_creator/190  "VINP_RrFailcodehistory2_enum"
  bus_selector_1/170 -> UnitConverter_191/1  "<VINP_RrLLCTemp_C>"
  UnitConverter_191/1 -> bus_creator/191  "VINP_RrLLCTemp_C"
  bus_selector_1/171 -> UnitConverter_192/1  "<VINP_RrLLCflowReq_Lpmin>"
  UnitConverter_192/1 -> bus_creator/192  "VINP_RrLLCflowReq_Lpmin"
  bus_selector_1/172 -> UnitConverter_193/1  "<VINP_RrMCU3HWVer_enum>"
  UnitConverter_193/1 -> bus_creator/193  "VINP_RrMCU3HWVer_enum"
  bus_selector_1/173 -> UnitConverter_194/1  "<VINP_RrMCU3SWVer_enum>"
  UnitConverter_194/1 -> bus_creator/194  "VINP_RrMCU3SWVer_enum"
  bus_selector_1/174 -> UnitConverter_195/1  "<VINP_RrMCUTempWarn_enum>"
  UnitConverter_195/1 -> bus_creator/195  "VINP_RrMCUTempWarn_enum"
  bus_selector_1/175 -> UnitConverter_196/1  "<VINP_RrTMTempWarn_enum>"
  UnitConverter_196/1 -> bus_creator/196  "VINP_RrTMTempWarn_enum"
  bus_selector_1/176 -> UnitConverter_197/1  "<VINP_MCUNF1CSErr_flg>"
  UnitConverter_197/1 -> bus_creator/197  "VINP_MCUNF1CSErr_flg"
  bus_selector_1/177 -> UnitConverter_198/1  "<VINP_MCUNF1RCErr_flg>"
  UnitConverter_198/1 -> bus_creator/198  "VINP_MCUNF1RCErr_flg"
  bus_selector_1/178 -> UnitConverter_199/1  "<VINP_FrActvDmpDisabStaNidec_flg>"
  UnitConverter_199/1 -> bus_creator/199  "VINP_FrActvDmpDisabStaNidec_flg"
  bus_selector_1/179 -> UnitConverter_200/1  "<VINP_FrEDUDrtStaNidec_flg>"
  UnitConverter_200/1 -> bus_creator/200  "VINP_FrEDUDrtStaNidec_flg"
  bus_selector_1/180 -> UnitConverter_201/1  "<VINP_FrEDUOpratingStaNidec_flg>"
  UnitConverter_201/1 -> bus_creator/201  "VINP_FrEDUOpratingStaNidec_flg"
  bus_selector_1/181 -> UnitConverter_202/1  "<VINP_FrEDURealTMTqNidec_Nm>"
  UnitConverter_202/1 -> bus_creator/202  "VINP_FrEDURealTMTqNidec_Nm"
  bus_selector_1/182 -> UnitConverter_203/1  "<VINP_FrEDURotateDirctionNidec_enum>"
  UnitConverter_203/1 -> bus_creator/203  "VINP_FrEDURotateDirctionNidec_enum"
  bus_selector_1/183 -> UnitConverter_204/1  "<VINP_FrEDUTqReqFbkNidec_Nm>"
  UnitConverter_204/1 -> bus_creator/204  "VINP_FrEDUTqReqFbkNidec_Nm"
  bus_selector_1/184 -> UnitConverter_205/1  "<VINP_FrMCU1ChksumNidec_enum>"
  UnitConverter_205/1 -> bus_creator/205  "VINP_FrMCU1ChksumNidec_enum"
  bus_selector_1/185 -> UnitConverter_206/1  "<VINP_FrMCU1RolCntNidec_enum>"
  UnitConverter_206/1 -> bus_creator/206  "VINP_FrMCU1RolCntNidec_enum"
  bus_selector_1/186 -> UnitConverter_207/1  "<VINP_FrMCUBATNidec_V>"
  UnitConverter_207/1 -> bus_creator/207  "VINP_FrMCUBATNidec_V"
  bus_selector_1/187 -> UnitConverter_208/1  "<VINP_FrMCUDCBusCurrNidec_A>"
  UnitConverter_208/1 -> bus_creator/208  "VINP_FrMCUDCBusCurrNidec_A"
  bus_selector_1/188 -> UnitConverter_209/1  "<VINP_FrMCUDCBusVoltNidec_V>"
  UnitConverter_209/1 -> bus_creator/209  "VINP_FrMCUDCBusVoltNidec_V"
  bus_selector_1/189 -> UnitConverter_210/1  "<VINP_FrMCUDischrgStaNidec_flg>"
  UnitConverter_210/1 -> bus_creator/210  "VINP_FrMCUDischrgStaNidec_flg"
  bus_selector_1/190 -> UnitConverter_211/1  "<VINP_FrMCUEnaStaNidec_flg>"
  UnitConverter_211/1 -> bus_creator/211  "VINP_FrMCUEnaStaNidec_flg"
  bus_selector_1/191 -> UnitConverter_212/1  "<VINP_FrMCUErrNidec_enum>"
  UnitConverter_212/1 -> bus_creator/212  "VINP_FrMCUErrNidec_enum"
  bus_selector_1/192 -> UnitConverter_213/1  "<VINP_FrMCUIGNstaNidec_flg>"
  UnitConverter_213/1 -> bus_creator/213  "VINP_FrMCUIGNstaNidec_flg"
  bus_selector_1/193 -> UnitConverter_214/1  "<VINP_FrMCUReady4PreNidec_flg>"
  UnitConverter_214/1 -> bus_creator/214  "VINP_FrMCUReady4PreNidec_flg"
  bus_selector_1/194 -> UnitConverter_215/1  "<VINP_FrMCUReadyNidec_flg>"
  UnitConverter_215/1 -> bus_creator/215  "VINP_FrMCUReadyNidec_flg"
  bus_selector_1/195 -> UnitConverter_216/1  "<VINP_FrMCUSysStaNidec_enum>"
  UnitConverter_216/1 -> bus_creator/216  "VINP_FrMCUSysStaNidec_enum"
  bus_selector_1/196 -> UnitConverter_217/1  "<VINP_FrMCUTempNidec_C>"
  UnitConverter_217/1 -> bus_creator/217  "VINP_FrMCUTempNidec_C"
  bus_selector_1/197 -> UnitConverter_218/1  "<VINP_FrMotorAvailTqNidec_Nm>"
  UnitConverter_218/1 -> bus_creator/218  "VINP_FrMotorAvailTqNidec_Nm"
  bus_selector_1/198 -> UnitConverter_219/1  "<VINP_FrRegenAvailTqNidec_Nm>"
  UnitConverter_219/1 -> bus_creator/219  "VINP_FrRegenAvailTqNidec_Nm"
  bus_selector_1/199 -> UnitConverter_220/1  "<VINP_FrTMSpdNidec_rpm>"
  UnitConverter_220/1 -> bus_creator/220  "VINP_FrTMSpdNidec_rpm"
  bus_selector_1/200 -> UnitConverter_221/1  "<VINP_FrTMTempNidec_C>"
  UnitConverter_221/1 -> bus_creator/221  "VINP_FrTMTempNidec_C"
  bus_selector_1/201 -> UnitConverter_222/1  "<VINP_FrTMidNidec_A>"
  UnitConverter_222/1 -> bus_creator/222  "VINP_FrTMidNidec_A"
  bus_selector_1/202 -> UnitConverter_223/1  "<VINP_FrTMiqNidec_A>"
  UnitConverter_223/1 -> bus_creator/223  "VINP_FrTMiqNidec_A"
  bus_selector_1/203 -> UnitConverter_224/1  "<VINP_MCUWarnFNidec_enum>"
  UnitConverter_224/1 -> bus_creator/224  "VINP_MCUWarnFNidec_enum"
  bus_selector_1/204 -> UnitConverter_225/1  "<VINP_FrCoolanttempReqNidec_C>"
  UnitConverter_225/1 -> bus_creator/225  "VINP_FrCoolanttempReqNidec_C"
  bus_selector_1/205 -> UnitConverter_226/1  "<VINP_FrEOPSpdSetNidec_rpm>"
  UnitConverter_226/1 -> bus_creator/226  "VINP_FrEOPSpdSetNidec_rpm"
  bus_selector_1/206 -> UnitConverter_227/1  "<VINP_FrFailcode1Nidec_enum>"
  UnitConverter_227/1 -> bus_creator/227  "VINP_FrFailcode1Nidec_enum"
  bus_selector_1/207 -> UnitConverter_228/1  "<VINP_FrFailcode2Nidec_enum>"
  UnitConverter_228/1 -> bus_creator/228  "VINP_FrFailcode2Nidec_enum"
  bus_selector_1/208 -> UnitConverter_229/1  "<VINP_FrFailcodehistory1Nidec_enum>"
  UnitConverter_229/1 -> bus_creator/229  "VINP_FrFailcodehistory1Nidec_enum"
  bus_selector_1/209 -> UnitConverter_230/1  "<VINP_FrFailcodehistory2Nidec_enum>"
  UnitConverter_230/1 -> bus_creator/230  "VINP_FrFailcodehistory2Nidec_enum"
  bus_selector_1/210 -> UnitConverter_231/1  "<VINP_FrLLCTempNidec_C>"
  UnitConverter_231/1 -> bus_creator/231  "VINP_FrLLCTempNidec_C"
  bus_selector_1/211 -> UnitConverter_232/1  "<VINP_FrLLCflowReqNidec_Lpmin>"
  UnitConverter_232/1 -> bus_creator/232  "VINP_FrLLCflowReqNidec_Lpmin"
  bus_selector_1/212 -> UnitConverter_233/1  "<VINP_FrMCUTempWarnNidec_enum>"
  UnitConverter_233/1 -> bus_creator/233  "VINP_FrMCUTempWarnNidec_enum"
  bus_selector_1/213 -> UnitConverter_234/1  "<VINP_FrTMTempWarnNidec_enum>"
  UnitConverter_234/1 -> bus_creator/234  "VINP_FrTMTempWarnNidec_enum"
  bus_selector_1/214 -> UnitConverter_235/1  "<VINP_FrMCUHWVerNidec_enum>"
  UnitConverter_235/1 -> bus_creator/235  "VINP_FrMCUHWVerNidec_enum"
  bus_selector_1/215 -> UnitConverter_236/1  "<VINP_FrMCUSWVerNidec_enum>"
  UnitConverter_236/1 -> bus_creator/236  "VINP_FrMCUSWVerNidec_enum"
  bus_selector_1/216 -> UnitConverter_237/1  "<VINP_MCUNR1CSErr_flg>"
  UnitConverter_237/1 -> bus_creator/237  "VINP_MCUNR1CSErr_flg"
  bus_selector_1/217 -> UnitConverter_238/1  "<VINP_MCUNR1RCErr_flg>"
  UnitConverter_238/1 -> bus_creator/238  "VINP_MCUNR1RCErr_flg"
  bus_selector_1/218 -> UnitConverter_239/1  "<VINP_MCUWarnRNidec_enum>"
  UnitConverter_239/1 -> bus_creator/239  "VINP_MCUWarnRNidec_enum"
  bus_selector_1/219 -> UnitConverter_240/1  "<VINP_RrActvDmpDisabStaNidec_flg>"
  UnitConverter_240/1 -> bus_creator/240  "VINP_RrActvDmpDisabStaNidec_flg"
  bus_selector_1/220 -> UnitConverter_241/1  "<VINP_RrEDUDrtStaNidec_flg>"
  UnitConverter_241/1 -> bus_creator/241  "VINP_RrEDUDrtStaNidec_flg"
  bus_selector_1/221 -> UnitConverter_242/1  "<VINP_RrEDUOpratingStaNidec_flg>"
  UnitConverter_242/1 -> bus_creator/242  "VINP_RrEDUOpratingStaNidec_flg"
  bus_selector_1/222 -> UnitConverter_243/1  "<VINP_RrEDURealTMTqNidec_Nm>"
  UnitConverter_243/1 -> bus_creator/243  "VINP_RrEDURealTMTqNidec_Nm"
  bus_selector_1/223 -> UnitConverter_244/1  "<VINP_RrEDURotateDirctionNidec_enum>"
  UnitConverter_244/1 -> bus_creator/244  "VINP_RrEDURotateDirctionNidec_enum"
  bus_selector_1/224 -> UnitConverter_245/1  "<VINP_RrEDUTqReqFbkNidec_Nm>"
  UnitConverter_245/1 -> bus_creator/245  "VINP_RrEDUTqReqFbkNidec_Nm"
  bus_selector_1/225 -> UnitConverter_246/1  "<VINP_RrMCU1ChksumNidec_enum>"
  UnitConverter_246/1 -> bus_creator/246  "VINP_RrMCU1ChksumNidec_enum"
  bus_selector_1/226 -> UnitConverter_247/1  "<VINP_RrMCU1RolCntNidec_enum>"
  UnitConverter_247/1 -> bus_creator/247  "VINP_RrMCU1RolCntNidec_enum"
  bus_selector_1/227 -> UnitConverter_248/1  "<VINP_RrMCUBATNidec_V>"
  UnitConverter_248/1 -> bus_creator/248  "VINP_RrMCUBATNidec_V"
  bus_selector_1/228 -> UnitConverter_249/1  "<VINP_RrMCUDCBusCurrNidec_A>"
  UnitConverter_249/1 -> bus_creator/249  "VINP_RrMCUDCBusCurrNidec_A"
  bus_selector_1/229 -> UnitConverter_250/1  "<VINP_RrMCUDCBusVoltNidec_V>"
  UnitConverter_250/1 -> bus_creator/250  "VINP_RrMCUDCBusVoltNidec_V"
  bus_selector_1/230 -> UnitConverter_251/1  "<VINP_RrMCUDischrgStaNidec_flg>"
  UnitConverter_251/1 -> bus_creator/251  "VINP_RrMCUDischrgStaNidec_flg"
  bus_selector_1/231 -> UnitConverter_252/1  "<VINP_RrMCUEnaStaNidec_flg>"
  UnitConverter_252/1 -> bus_creator/252  "VINP_RrMCUEnaStaNidec_flg"
  bus_selector_1/232 -> UnitConverter_253/1  "<VINP_RrMCUErrNidec_enum>"
  UnitConverter_253/1 -> bus_creator/253  "VINP_RrMCUErrNidec_enum"
  bus_selector_1/233 -> UnitConverter_254/1  "<VINP_RrMCUIGNstaNidec_flg>"
  UnitConverter_254/1 -> bus_creator/254  "VINP_RrMCUIGNstaNidec_flg"
  bus_selector_1/234 -> UnitConverter_255/1  "<VINP_RrMCUReady4PreNidec_flg>"
  UnitConverter_255/1 -> bus_creator/255  "VINP_RrMCUReady4PreNidec_flg"
  bus_selector_1/235 -> UnitConverter_256/1  "<VINP_RrMCUReadyNidec_flg>"
  UnitConverter_256/1 -> bus_creator/256  "VINP_RrMCUReadyNidec_flg"
  bus_selector_1/236 -> UnitConverter_257/1  "<VINP_RrMCUSysStaNidec_enum>"
  UnitConverter_257/1 -> bus_creator/257  "VINP_RrMCUSysStaNidec_enum"
  bus_selector_1/237 -> UnitConverter_258/1  "<VINP_RrMCUTempNidec_C>"
  UnitConverter_258/1 -> bus_creator/258  "VINP_RrMCUTempNidec_C"
  bus_selector_1/238 -> UnitConverter_259/1  "<VINP_RrMotorAvailTqNidec_Nm>"
  UnitConverter_259/1 -> bus_creator/259  "VINP_RrMotorAvailTqNidec_Nm"
  bus_selector_1/239 -> UnitConverter_260/1  "<VINP_RrRegenAvailTqNidec_Nm>"
  UnitConverter_260/1 -> bus_creator/260  "VINP_RrRegenAvailTqNidec_Nm"
  bus_selector_1/240 -> UnitConverter_261/1  "<VINP_RrTMSpdNidec_rpm>"
  UnitConverter_261/1 -> bus_creator/261  "VINP_RrTMSpdNidec_rpm"
  bus_selector_1/241 -> UnitConverter_262/1  "<VINP_RrTMTempNidec_C>"
  UnitConverter_262/1 -> bus_creator/262  "VINP_RrTMTempNidec_C"
  bus_selector_1/242 -> UnitConverter_263/1  "<VINP_RrTMidNidec_A>"
  UnitConverter_263/1 -> bus_creator/263  "VINP_RrTMidNidec_A"
  bus_selector_1/243 -> UnitConverter_264/1  "<VINP_RrTMiqNidec_A>"
  UnitConverter_264/1 -> bus_creator/264  "VINP_RrTMiqNidec_A"
  bus_selector_1/244 -> UnitConverter_265/1  "<VINP_RrCoolanttempReqNidec_cnt>"
  UnitConverter_265/1 -> bus_creator/265  "VINP_RrCoolanttempReqNidec_cnt"
  bus_selector_1/245 -> UnitConverter_266/1  "<VINP_RrEOPSpdSetNidec_rpm>"
  UnitConverter_266/1 -> bus_creator/266  "VINP_RrEOPSpdSetNidec_rpm"
  bus_selector_1/246 -> UnitConverter_267/1  "<VINP_RrFailcode1Nidec_enum>"
  UnitConverter_267/1 -> bus_creator/267  "VINP_RrFailcode1Nidec_enum"
  bus_selector_1/247 -> UnitConverter_268/1  "<VINP_RrFailcode2Nidec_enum>"
  UnitConverter_268/1 -> bus_creator/268  "VINP_RrFailcode2Nidec_enum"
  bus_selector_1/248 -> UnitConverter_269/1  "<VINP_RrFailcodehistory1Nidec_enum>"
  UnitConverter_269/1 -> bus_creator/269  "VINP_RrFailcodehistory1Nidec_enum"
  bus_selector_1/249 -> UnitConverter_270/1  "<VINP_RrFailcodehistory2Nidec_enum>"
  UnitConverter_270/1 -> bus_creator/270  "VINP_RrFailcodehistory2Nidec_enum"
  bus_selector_1/250 -> UnitConverter_271/1  "<VINP_RrLLCTempNidec_C>"
  UnitConverter_271/1 -> bus_creator/271  "VINP_RrLLCTempNidec_C"
  bus_selector_1/251 -> UnitConverter_272/1  "<VINP_RrLLCflowReqNidec_Lpmin>"
  UnitConverter_272/1 -> bus_creator/272  "VINP_RrLLCflowReqNidec_Lpmin"
  bus_selector_1/252 -> UnitConverter_273/1  "<VINP_RrMCUTempWarnNidec_enum>"
  UnitConverter_273/1 -> bus_creator/273  "VINP_RrMCUTempWarnNidec_enum"
  bus_selector_1/253 -> UnitConverter_274/1  "<VINP_RrTMTempWarnNidec_enum>"
  UnitConverter_274/1 -> bus_creator/274  "VINP_RrTMTempWarnNidec_enum"
  bus_selector_1/254 -> UnitConverter_275/1  "<VINP_RrMCU3HWVerNidec_enum>"
  UnitConverter_275/1 -> bus_creator/275  "VINP_RrMCU3HWVerNidec_enum"
  bus_selector_1/255 -> UnitConverter_276/1  "<VINP_RrMCU3SWVerNidec_enum>"
  UnitConverter_276/1 -> bus_creator/276  "VINP_RrMCU3SWVerNidec_enum"
  bus_selector_1/256 -> UnitConverter_277/1  "<VINP_Shifter1CSErr_flg>"
  UnitConverter_277/1 -> bus_creator/277  "VINP_Shifter1CSErr_flg"
  bus_selector_1/257 -> UnitConverter_278/1  "<VINP_Shifter1RCErr_flg>"
  UnitConverter_278/1 -> bus_creator/278  "VINP_Shifter1RCErr_flg"
  bus_selector_1/258 -> UnitConverter_279/1  "<VINP_ShifterCRC8_enum>"
  UnitConverter_279/1 -> bus_creator/279  "VINP_ShifterCRC8_enum"
  bus_selector_1/259 -> UnitConverter_280/1  "<VINP_ShifterFailsta_enum>"
  UnitConverter_280/1 -> bus_creator/280  "VINP_ShifterFailsta_enum"
  bus_selector_1/260 -> UnitConverter_281/1  "<VINP_ShifterHandleCmd_enum>"
  UnitConverter_281/1 -> bus_creator/281  "VINP_ShifterHandleCmd_enum"
  bus_selector_1/261 -> UnitConverter_282/1  "<VINP_ShifterRC_enum>"
  UnitConverter_282/1 -> bus_creator/282  "VINP_ShifterRC_enum"
  bus_selector_1/262 -> UnitConverter_283/1  "<VINP_Shifter2CSErr_flg>"
  UnitConverter_283/1 -> bus_creator/283  "VINP_Shifter2CSErr_flg"
  bus_selector_1/263 -> UnitConverter_284/1  "<VINP_Shifter2RCErr_flg>"
  UnitConverter_284/1 -> bus_creator/284  "VINP_Shifter2RCErr_flg"
  bus_selector_1/264 -> UnitConverter_285/1  "<VINP_CSW2DimSwSta_flg>"
  UnitConverter_285/1 -> bus_creator/285  "VINP_CSW2DimSwSta_flg"
  bus_selector_1/265 -> UnitConverter_286/1  "<VINP_CSW2FWasSwSta_enum>"
  UnitConverter_286/1 -> bus_creator/286  "VINP_CSW2FWasSwSta_enum"
  bus_selector_1/266 -> UnitConverter_287/1  "<VINP_CSW2FWipSwSta_enum>"
  UnitConverter_287/1 -> bus_creator/287  "VINP_CSW2FWipSwSta_enum"
  bus_selector_1/267 -> UnitConverter_288/1  "<VINP_CSW2PassSWSta_flg>"
  UnitConverter_288/1 -> bus_creator/288  "VINP_CSW2PassSWSta_flg"
  bus_selector_1/268 -> UnitConverter_289/1  "<VINP_CSW2RWipWasSwSta_enum>"
  UnitConverter_289/1 -> bus_creator/289  "VINP_CSW2RWipWasSwSta_enum"
  bus_selector_1/269 -> UnitConverter_290/1  "<VINP_CSW2TurnSwSta_enum>"
  UnitConverter_290/1 -> bus_creator/290  "VINP_CSW2TurnSwSta_enum"
  [inp_CanValid_bus] -> bus_selector/1
  [inp_Hal_bus] -> bus_selector_1/1
  bus_creator/1 -> BINP_outputs/1
